simulink model "QUESTION4_23"  (R2021a)
settings: Solver=VariableStepAuto  StartTime=0.0  StopTime=200  RelTol=1e-3
settings Model: Creator=user  LastModifiedBy=user

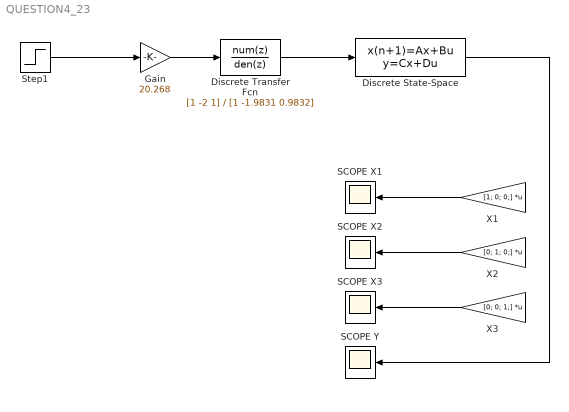
== system QUESTION4_23 ==
  Discrete Transfer Fcn : DiscreteTransferFcn  Numerator=[1 -2 1]  Denominator=[1 -1.9831 0.9832]
  Discrete State-Space : DiscreteStateSpace  A=|  B=|  C=[0 0 1]  D=0  SampleTime=0.5
      A=|
      | [0.8796    0.4676   -0.4676;
      |    -0.4209    0.8495    0.1505;
      |     0.0468    0.0167    0.9833;]
      B=|
      | [0.1084;
      |     0.4238;
      |     0.0029;]
  Gain : Gain  Gain=20.268
  SCOPE X1 : Scope
  SCOPE X2 : Scope
  SCOPE X3 : Scope
  SCOPE Y : Scope
  Step1 : Step  SampleTime=0
  X1 : Gain  Gain=[1; 0; 0;]  Multiplication=Matrix(K*u)
  X2 : Gain  Gain=[0; 1; 0;]  Multiplication=Matrix(K*u)
  X3 : Gain  Gain=[0; 0; 1;]  Multiplication=Matrix(K*u)
  wires:
  X1/1 -> SCOPE X1/1
  X2/1 -> SCOPE X2/1
  X3/1 -> SCOPE X3/1
  Discrete State-Space/1 -> SCOPE Y/1
  Step1/1 -> Gain/1
  Discrete Transfer Fcn/1 -> Discrete State-Space/1
  Gain/1 -> Discrete Transfer Fcn/1
